simulink model "bluetooth"  (R2020a)
settings: Solver=FixedStepAuto  StartTime=0.0  StopTime=10.0  RelTol=1e-3
undefined symbols (not defined in the file): BC, Ci, Ri, tau1
libraries: androiduilib x12, simulink x5, androidcommunicationlib x2, dspswit3 x2
settings Model: Creator=luisi  LastModifiedBy=luisi
settings OptimizationCC: EnhancedBackFolding=on  PassReuseOutputArgsAs=Individual arguments  ZeroExternalMemoryAtStartup=off  ZeroInternalMemoryAtStartup=off  MaxStackSize=64  OptimizeBlockOrder=speed  DifferentSizesBufferReuse=on  OptimizationCustomize=off  EfficientTunableParamExpr=on
settings DebuggingCC: ParameterTunabilityLossMsg=error
settings HardwareCC: ProdBitPerPointer=32  ProdBitPerSizeT=32  ProdBitPerPtrDiffT=32  ProdLargestAtomicInteger=Long  ProdLargestAtomicFloat=Double  ProdWordSize=32  ProdHWDeviceType=ARM Compatible->ARM Cortex
settings SFSimCC: MATLABDynamicMemAlloc=off
settings RTWCC: SystemTargetFile=ert.tlc  HardwareBoard=Android Device  TemplateMakefile=ert_default_tmf  RTWVerbose=off  Toolchain=Android SDK/NDK Tools
settings CodeAppCC: ForceParamTrailComments=on  IgnoreCustomStorageClasses=off  OperatorAnnotations=on  SimulinkDataObjDesc=on  SFDataObjDesc=on  InsertBlockDesc=on
settings ERTTargetCC: SupportContinuousTime=on  SupportVariableSizeSignals=on  ExtModeMexArgs='192.168.0.149'

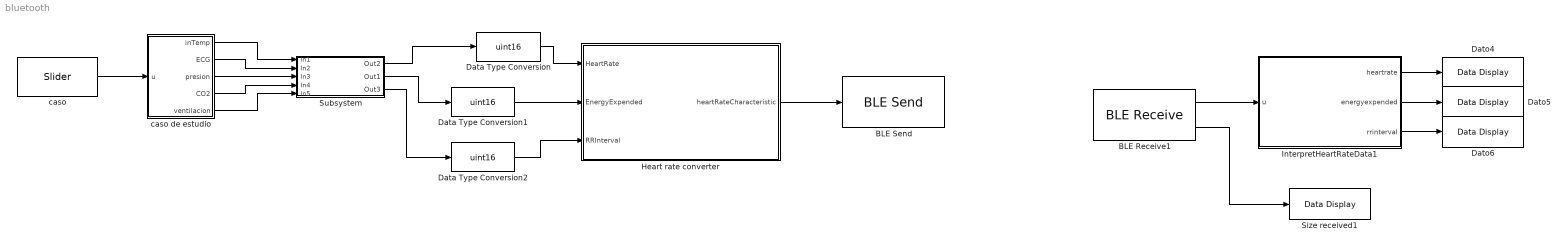
== system bluetooth ==
  BLE Receive1 : androidcommunicationlib/BLE Receive  DeviceMode=Central (Client)  BluetoothAddress=75:BC:6F:E0:E0:E0  CharUUID=00002a37-0000-1000-8000-00805f9b34fb  ServiceUUID=0000180d-0000-1000-8000-00805f9b34fb  device=RedmiMama  character="Heart Rate\\Heart Rate  Measurement"  CustomService=off  ServiceName=Heart Rate  CharacteristicName="Heart Rate  Measurement"  CustomServiceUUID=<Enter Service UUID>  CustomCharUUID=<Enter Characteristic UUID>  DataSize=7  SampleTime=0.1  charseruuid=00001801-0000-1000-8000-00805f9b34fb\00002a05-0000-1000-8000-00805f9b34fb  seruuid=00001810-0000-1000-8000-00805f9b34fb  PeripheralService=0000180d-0000-1000-8000-00805f9b34fb  PeripheralCharacteristic=00002a37-0000-1000-8000-00805f9b34fb  chruuid=00002a37-0000-1000-8000-00805f9b34fb  BLEId=bluetooth/BLE_Receive1  Devicename=RedmiMama  IsCustomService=0
      settings: SourceProductBaseCode=ANDROID
  BLE Send : androidcommunicationlib/BLE Send  DeviceMode=Peripheral (Server)  BluetoothAddress=75:BC:6F:E0:E0:E0  CharUUID=00002a05-0000-1000-8000-00805f9b34fb  ServiceUUID=00001801-0000-1000-8000-00805f9b34fb  device=RedmiMama  character=Generic Attribute\Service Changed  CustomService=off  ServiceName=Heart Rate  CharacteristicName="Heart Rate  Measurement"  CustomServiceUUID=<Enter Service UUID>  CustomCharUUID=<Enter Characteristic UUID>  charseruuid=00001801-0000-1000-8000-00805f9b34fb\00002a05-0000-1000-8000-00805f9b34fb  seruuid=00001810-0000-1000-8000-00805f9b34fb  chruuid=00002a37-0000-1000-8000-00805f9b34fb  PeripheralService=0000180d-0000-1000-8000-00805f9b34fb  PeripheralCharacteristic=00002a37-0000-1000-8000-00805f9b34fb  BLEId=bluetooth/BLE_Send  Devicename=RedmiMama  IsCustomService=0  Size=-1
      settings: SourceProductBaseCode=ANDROID
  Data Type Conversion : DataTypeConversion  OutDataTypeStr=uint16
  Data Type Conversion1 : DataTypeConversion  OutDataTypeStr=uint16
  Data Type Conversion2 : DataTypeConversion  OutDataTypeStr=uint16
  Dato4 : androiduilib/Data Display  DataDisplayId=bluetooth/Dato4  Format=Float  Precision=6  SimulateUsing=Code generation  blockPlatform=Android
      settings: SourceProductBaseCode=ANDROID
  Dato5 : androiduilib/Data Display  DataDisplayId=bluetooth/Dato5  Format=Float  Precision=6  SimulateUsing=Code generation  blockPlatform=Android
      settings: SourceProductBaseCode=ANDROID
  Dato6 : androiduilib/Data Display  DataDisplayId=bluetooth/Dato6  Format=Float  Precision=6  SimulateUsing=Code generation  blockPlatform=Android
      settings: SourceProductBaseCode=ANDROID
  Heart rate converter : MATLAB Function  TreatAsAtomicUnit=on
  InterpretHeartRateData1 : MATLAB Function  TreatAsAtomicUnit=on
  Size received1 : androiduilib/Data Display  DataDisplayId=bluetooth/Size_received1  Format=Float  Precision=6  SimulateUsing=Code generation  blockPlatform=Android
      settings: SourceProductBaseCode=ANDROID
  Subsystem : Subsystem
  caso : androiduilib/Slider  Min=0  Value=0  Max=2  Resolution=1  SliderId=bluetooth/caso  SampleTime=0.01  BlockPlatform=Android
      settings: SourceProductBaseCode=ANDROID
  caso de estudio : MATLAB Function  TreatAsAtomicUnit=on
  wires:
  Data Type Conversion2/1 -> Heart rate converter/3(RRInterval)
  Heart rate converter/1(heartRateCharacteristic) -> BLE Send/1
  Data Type Conversion/1 -> Heart rate converter/1(HeartRate)
  Data Type Conversion1/1 -> Heart rate converter/2(EnergyExpended)
  Subsystem/1(Out2) -> Data Type Conversion/1
  Subsystem/2(Out1) -> Data Type Conversion1/1
  Subsystem/3(Out3) -> Data Type Conversion2/1
  InterpretHeartRateData1/1(heartrate) -> Dato4/1
  BLE Receive1/2 -> Size received1/1
  InterpretHeartRateData1/2(energyexpended) -> Dato5/1
  InterpretHeartRateData1/3(rrinterval) -> Dato6/1
  BLE Receive1/1 -> InterpretHeartRateData1/1(u)
  caso de estudio/3(presion) -> Subsystem/3(In3)
  caso/1 -> caso de estudio/1(u)
  caso de estudio/4(CO2) -> Subsystem/4(In4)
  caso de estudio/2(ECG) -> Subsystem/2(In2)
  caso de estudio/5(ventilacion) -> Subsystem/5(In5)
  caso de estudio/1(inTemp) -> Subsystem/1(In1)

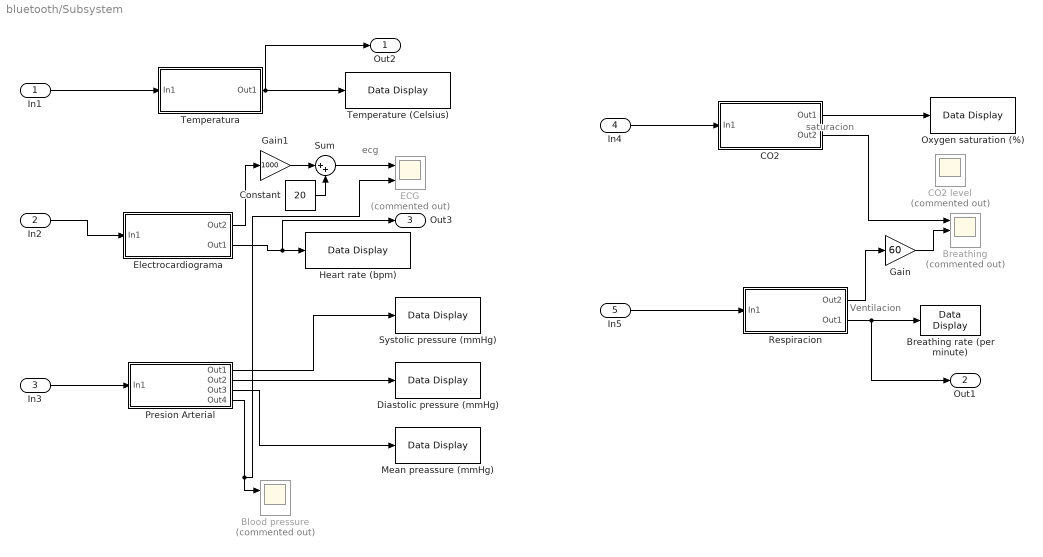
== system bluetooth/Subsystem ==
  note: ecg
  note: saturacion
  note: Ventilacion
  In1 : Inport
  In2 : Inport  Port=2
  In3 : Inport  Port=3
  In4 : Inport  Port=4
  In5 : Inport  Port=5
  Blood pressure : Scope  Commented=on  NumInputPorts=2
  Breathing : Scope  Commented=on  NumInputPorts=3
  Breathing rate (per minute) : androiduilib/Data Display  DataDisplayId=bluetooth/Subsystem/Breathing_rate_(per_minute)  Format=Integer  Precision=6  SimulateUsing=Code generation  blockPlatform=Android
      settings: SourceProductBaseCode=ANDROID
  CO2 : Subsystem
  "CO2 level " : Scope  Commented=on
  Constant : Constant  Value=20
  Diastolic pressure (mmHg) : androiduilib/Data Display  DataDisplayId=bluetooth/Subsystem/Diastolic_pressure_(mmHg)  Format=Integer  Precision=6  SimulateUsing=Code generation  blockPlatform=Android
      settings: SourceProductBaseCode=ANDROID
  ECG : Scope  Commented=on  NumInputPorts=2
      settings: AttributesFormatString=%<AxesScaling>
  Electrocardiograma : Subsystem
  Gain : Gain  Gain=60
  Gain1 : Gain  Gain=1000
  Heart rate (bpm) : androiduilib/Data Display  DataDisplayId=bluetooth/Subsystem/Heart_rate_(bpm)  Format=Float  Precision=6  SimulateUsing=Code generation  blockPlatform=Android
      settings: SourceProductBaseCode=ANDROID
  Mean preassure (mmHg) : androiduilib/Data Display  DataDisplayId=bluetooth/Subsystem/Mean_preassure_(mmHg)  Format=Integer  Precision=6  SimulateUsing=Code generation  blockPlatform=Android
      settings: SourceProductBaseCode=ANDROID
  Oxygen saturation (%) : androiduilib/Data Display  DataDisplayId=bluetooth/Subsystem/Oxygen_saturation_(%)  Format=Integer  Precision=6  SimulateUsing=Code generation  blockPlatform=Android
      settings: SourceProductBaseCode=ANDROID
  Presion Arterial : Subsystem
  Respiracion : Subsystem
  Sum : Sum  Inputs=|++
  Systolic pressure (mmHg) : androiduilib/Data Display  DataDisplayId=bluetooth/Subsystem/Systolic_pressure_(mmHg)  Format=Integer  Precision=6  SimulateUsing=Code generation  blockPlatform=Android
      settings: SourceProductBaseCode=ANDROID
  Temperatura : Subsystem
  Temperature (Celsius) : androiduilib/Data Display  DataDisplayId=bluetooth/Subsystem/Temperature_(Celsius)  Format=Float  Precision=1  SimulateUsing=Code generation  blockPlatform=Android
      settings: SourceProductBaseCode=ANDROID
  Out2 : Outport
  Out1 : Outport  Port=2
  Out3 : Outport  Port=3
  wires:
  In1/1 -> Temperatura/1(In1)
  In2/1 -> Electrocardiograma/1(In1)
  Temperatura/1(Out1) -> Out2/1, Temperature (Celsius)/1
  Presion Arterial/2(Out2) -> Diastolic pressure (mmHg)/1
  Presion Arterial/3(Out3) -> Mean preassure (mmHg)/1
  Presion Arterial/1(Out1) -> Systolic pressure (mmHg)/1
  In5/1 -> Respiracion/1(In1)
  In3/1 -> Presion Arterial/1(In1)
  In4/1 -> CO2/1(In1)
  CO2/1(Out1) -> Oxygen saturation (%)/1
  Respiracion/2(Out1) -> Out1/1, Breathing rate (per minute)/1
  Electrocardiograma/2(Out1) -> Out3/1, Heart rate (bpm)/1
  CO2/2(Out2) -> Breathing/1
  Respiracion/1(Out2) -> Gain/1
  Gain/1 -> Breathing/2
  Presion Arterial/4(Out4) -> ECG/2, Blood pressure/1
  Electrocardiograma/1(Out2) -> Gain1/1
  Gain1/1 -> Sum/1
  Constant/1 -> Sum/2
  Sum/1 -> ECG/1

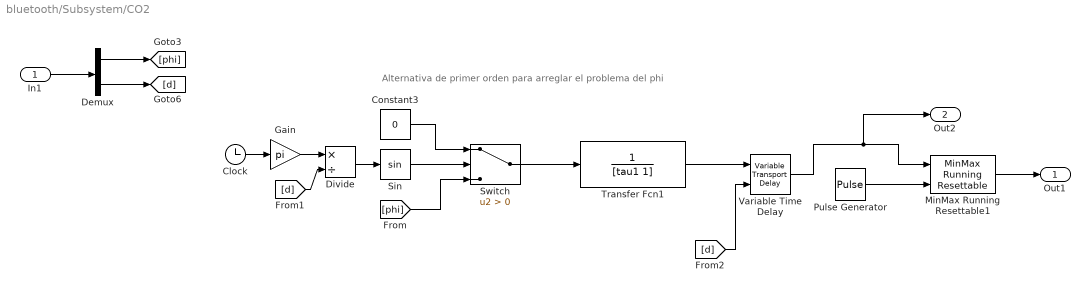
== system bluetooth/Subsystem/CO2 ==
  note: Alternativa de primer orden para arreglar el problema del phi
  In1 : Inport
  Clock : Clock
  Constant3 : Constant  Value=0
  Demux : Demux  Outputs=2
  Divide : Product  Inputs=*/
  Gain : Gain  Gain=pi
  MinMax Running Resettable1 : simulink/Math Operations/MinMax Running Resettable  Function=max  vinit=0
  Pulse Generator : DiscretePulseGenerator  PulseType=Time based  Period=4  PulseWidth=5  PhaseDelay=0.01
  Sin : Trigonometry
  Switch : Switch  Criteria=u2 > Threshold
  Transfer Fcn1 : TransferFcn  Denominator=[tau1 1]
  Variable Time Delay : VariableTransportDelay  MaximumDelay=10
  Out1 : Outport
  Out2 : Outport  Port=2
  wires:
  In1/1 -> Demux/1
  Demux/1 -> [phi]
  Switch/1 -> Transfer Fcn1/1
  Sin/1 -> Switch/2
  [phi] -> Switch/3
  Constant3/1 -> Switch/1
  Demux/2 -> [d]
  Clock/1 -> Gain/1
  Gain/1 -> Divide/1
  Divide/1 -> Sin/1
  [d] -> Divide/2
  MinMax Running Resettable1/1 -> Out1/1
  Pulse Generator/1 -> MinMax Running Resettable1/2
  Transfer Fcn1/1 -> Variable Time Delay/1
  Variable Time Delay/1 -> Out2/1, MinMax Running Resettable1/1
  [d] -> Variable Time Delay/2

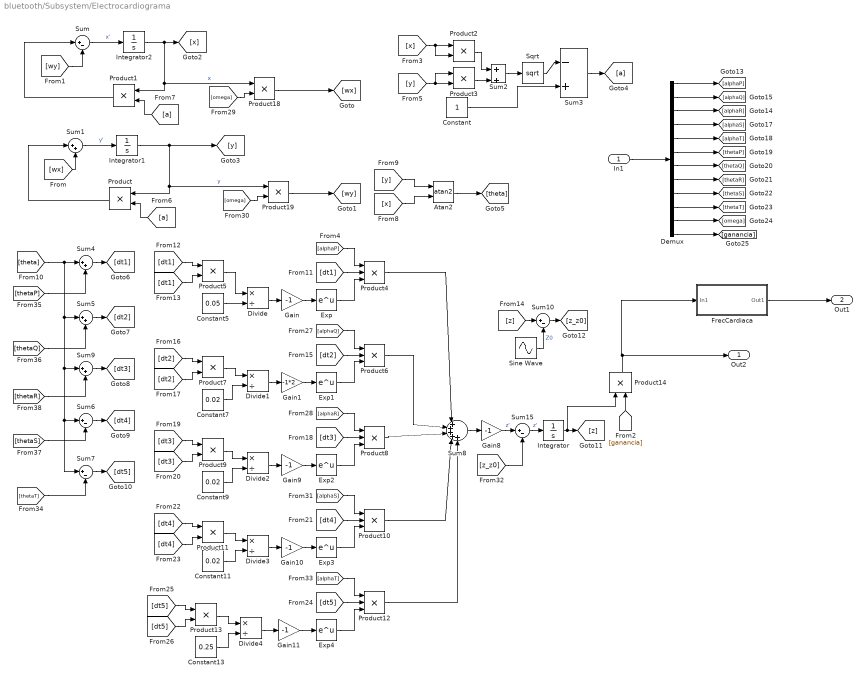
== system bluetooth/Subsystem/Electrocardiograma ==
  In1 : Inport
  Atan2 : Trigonometry  Operator=atan2
  Constant : Constant
  Constant11 : Constant  Value=0.02
  Constant13 : Constant  Value=0.25
  Constant5 : Constant  Value=0.05
  Constant7 : Constant  Value=0.02
  Constant9 : Constant  Value=0.02
  Demux : Demux  Outputs=12
  Divide{,1..4} (5 alike) : Product  Inputs=*/
  Exp{,1..4} (5 alike) : Math  SaturateOnIntegerOverflow=on
  FrecCardiaca : Subsystem
  Gain{,8..11} (5 alike) : Gain  Gain=-1
  Gain1 : Gain  Gain=-1*2
  Integrator : Integrator  InitialCondition=1000
  Integrator1 : Integrator
  Integrator2 : Integrator  InitialCondition=2
  Product{,1..3,5,7,9,11,13..14,18..19} (12 alike) : Product
  Product{4,6,8,10,12} (5 alike) : Product  Inputs=3
  Sine Wave : Sin  Amplitude=0.15e-3  Frequency=0.25  SampleTime=0
  Sqrt : Sqrt  SaturateOnIntegerOverflow=on
  Sum{,6..7,10,15} (5 alike) : Sum  Inputs=|+-
  Sum{1..2,4..5,9} (5 alike) : Sum  Inputs=|++
  Sum3 : Sum  Inputs=|-+
  Sum8 : Sum  Inputs=|+++++
  Out2 : Outport
  Out1 : Outport  Port=2
  wires:
  [dt2] -> Product6/2
  Product4/1 -> Sum8/1
  [x] -> Atan2/2
  Product3/1 -> Sum2/2
  [y] -> Atan2/1
  FrecCardiaca/1(Out1) -> Out1/1
  Product/1 -> Sum1/1
  Product5/1 -> Divide/1
  [dt2] -> Product7/2
  Gain/1 -> Exp/1
  Product1/1 -> Sum/1
  Constant/1 -> Sum3/2
  Divide1/1 -> Gain1/1
  Exp4/1 -> Product12/3
  Exp3/1 -> Product10/3
  Gain11/1 -> Exp4/1
  Exp/1 -> Product4/3
  [alphaT] -> Product12/1
  Constant11/1 -> Divide3/2
  Divide2/1 -> Gain9/1
  [dt1] -> Product4/2
  Product18/1 -> [wx]
  Sum2/1 -> Sqrt/1
  [a] -> Product1/2
  [thetaP] -> Sum4/2
  Product8/1 -> Sum8/3
  Exp2/1 -> Product8/3
  Product11/1 -> Divide3/1
  [dt3] -> Product9/2
  Integrator1/1 -> [y], Product19/1, Product/1  "y"
  Constant5/1 -> Divide/2
  Product7/1 -> Divide1/1
  [dt4] -> Product11/1
  Sqrt/1 -> Sum3/1
  Product13/1 -> Divide4/1
  Gain10/1 -> Exp3/1
  [dt1] -> Product5/1
  Gain1/1 -> Exp1/1
  [dt5] -> Product13/2
  [dt4] -> Product11/2
  [dt1] -> Product5/2
  Constant9/1 -> Divide2/2
  [dt5] -> Product12/2
  Divide/1 -> Gain/1
  Divide4/1 -> Gain11/1
  [dt5] -> Product13/1
  Product12/1 -> Sum8/5
  Product6/1 -> Sum8/2
  Constant13/1 -> Divide4/2
  Product10/1 -> Sum8/4
  Sum5/1 -> [dt2]
  [dt4] -> Product10/2
  Sine Wave/1 -> Sum10/2  "Z0"
  Sum6/1 -> [dt4]
  Sum1/1 -> Integrator1/1  "y'"
  [dt3] -> Product9/1
  Atan2/1 -> [theta]
  [omega] -> Product19/2
  Sum7/1 -> [dt5]
  Sum10/1 -> [z_z0]
  Gain8/1 -> Sum15/1  "z'"
  Integrator/1 -> Product14/1, [z]
  [dt3] -> Product8/2
  [theta] -> Sum7/1, Sum6/1, Sum9/1, Sum5/1, Sum4/1
  [z_z0] -> Sum15/2
  [a] -> Product/2
  Integrator2/1 -> [x], Product1/1, Product18/1  "x"
  Exp1/1 -> Product6/3
  [thetaS] -> Sum6/2
  Sum4/1 -> [dt1]
  [alphaP] -> Product4/1
  Sum15/1 -> Integrator/1  "z'"
  Product19/1 -> [wy]
  Sum/1 -> Integrator2/1  "x'"
  [wx] -> Sum1/2
  [thetaT] -> Sum7/2
  [y] -> Product3/1, Product3/2
  [wy] -> Sum/2
  [thetaQ] -> Sum5/2
  Product9/1 -> Divide2/1
  Constant7/1 -> Divide1/2
  Sum3/1 -> [a]
  [x] -> Product2/2, Product2/1
  [dt2] -> Product7/1
  [z] -> Sum10/1
  Gain9/1 -> Exp2/1
  [omega] -> Product18/2
  Product2/1 -> Sum2/1
  Product14/1 -> FrecCardiaca/1(In1), Out2/1
  Divide3/1 -> Gain10/1
  Sum8/1 -> Gain8/1
  In1/1 -> Demux/1
  Demux/1 -> [alphaP]
  Demux/2 -> [alphaQ]
  Demux/3 -> [alphaR]
  Demux/4 -> [alphaS]
  Demux/5 -> [alphaT]
  Demux/6 -> [thetaP]
  Demux/7 -> [thetaQ]
  Demux/8 -> [thetaR]
  Demux/9 -> [thetaS]
  Demux/10 -> [thetaT]
  Demux/11 -> [omega]
  Demux/12 -> [ganancia]
  [ganancia] -> Product14/2
  [alphaS] -> Product10/1
  [alphaR] -> Product8/1
  [alphaQ] -> Product6/1
  Sum9/1 -> [dt3]
  [thetaR] -> Sum9/2

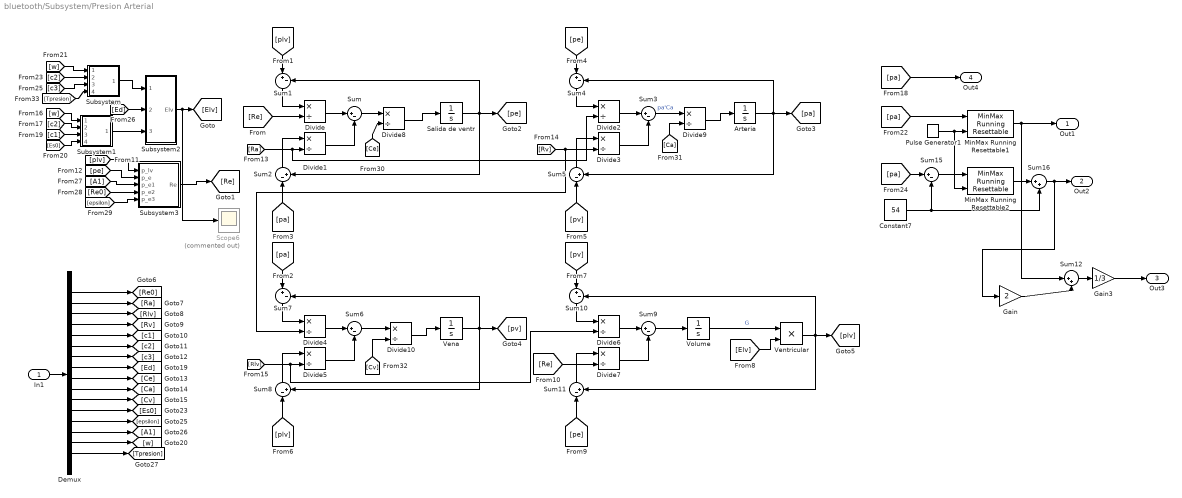
== system bluetooth/Subsystem/Presion Arterial ==
  In1 : Inport
  Arteria : Integrator  InitialCondition=70
  Constant7 : Constant  Value=54
  Demux : Demux  Outputs=16
  Divide{,1..10} (11 alike) : Product  Inputs=*/
  Gain : Gain  Gain=2
  Gain3 : Gain  Gain=1/3
  MinMax Running Resettable1 : simulink/Math Operations/MinMax Running Resettable  Function=max  vinit=40
  MinMax Running Resettable2 : simulink/Math Operations/MinMax Running Resettable  Function=min  vinit=0.0
  Pulse Generator1 : DiscretePulseGenerator  PulseType=Time based  Period=8  PulseWidth=5
  Salida de ventr : Integrator  InitialCondition=49.896
  Scope6 : Scope  Commented=on
  Subsystem : Subsystem
  Subsystem1 : Subsystem
  Subsystem2 : Subsystem
  Subsystem3 : Subsystem
  Sum{,1,3..4,6..7,9..10,15} (9 alike) : Sum  Inputs=|+-
  Sum{2,5,8,11} (4 alike) : Sum  Inputs=|-+
  Sum12 : Sum  Inputs=|++
  Sum16 : Sum  Inputs=|++
  Vena : Integrator  InitialCondition=16.628
  Ventricular : Product
  Volume : Integrator  InitialCondition=49.714/0.0655
  Out1 : Outport
  Out2 : Outport  Port=2
  Out3 : Outport  Port=3
  Out4 : Outport  Port=4
  wires:
  Gain3/1 -> Out3/1
  Sum16/1 -> Gain/1, Out2/1
  MinMax Running Resettable2/1 -> Sum16/1
  Sum3/1 -> Divide9/1  "pa'Ca"
  [pa] -> MinMax Running Resettable1/1
  Sum10/1 -> Divide6/1
  MinMax Running Resettable1/1 -> Sum12/1, Out1/1
  Subsystem2/1(Elv) -> Scope6/1, [Elv]
  Constant7/1 -> Sum16/2, Sum15/2
  Salida de ventr/1 -> [pe], Sum2/2, Sum1/2
  [pa] -> Sum15/1
  Divide6/1 -> Sum9/1
  Pulse Generator1/1 -> MinMax Running Resettable2/2, MinMax Running Resettable1/2
  [Elv] -> Ventricular/2
  [pa] -> Out4/1
  Divide8/1 -> Salida de ventr/1
  [Re] -> Divide/2
  [Rv] -> Divide4/2, Divide3/2
  Sum5/1 -> Divide3/1
  [plv] -> Subsystem3/1(p_lv)
  Divide/1 -> Sum/1
  [plv] -> Sum1/1
  [pv] -> Sum10/1
  Ventricular/1 -> Sum10/2, [plv], Sum11/2
  Sum15/1 -> MinMax Running Resettable2/1
  [pe] -> Sum4/1
  [pe] -> Subsystem3/2(p_e)
  Sum9/1 -> Volume/1
  [plv] -> Sum8/1
  Divide10/1 -> Vena/1
  [pv] -> Sum5/1
  Divide7/1 -> Sum9/2
  [Rlv] -> Divide6/2, Divide5/2
  Divide9/1 -> Arteria/1
  Sum8/1 -> Divide5/1
  Sum11/1 -> Divide7/1
  Divide2/1 -> Sum3/1
  [pe] -> Sum11/1
  [pa] -> Sum7/1
  Sum7/1 -> Divide4/1
  Vena/1 -> [pv], Sum8/2, Sum7/2
  Divide3/1 -> Sum3/2
  Sum6/1 -> Divide10/1
  Volume/1 -> Ventricular/1  "G"
  Divide5/1 -> Sum6/2
  Divide4/1 -> Sum6/1
  Arteria/1 -> Sum5/2, Sum4/2, [pa]
  [pa] -> Sum2/1
  [Re] -> Divide7/2
  Sum2/1 -> Divide1/1
  Sum1/1 -> Divide/1
  Sum/1 -> Divide8/1
  Sum4/1 -> Divide2/1
  Subsystem3/1(Re) -> [Re]
  Subsystem/1(alpha_t) -> Subsystem2/1(alpha)
  Subsystem1/1(E_s) -> Subsystem2/3(E_s)
  Divide1/1 -> Sum/2
  [Ra] -> Divide2/2, Divide1/2
  In1/1 -> Demux/1
  [w] -> Subsystem1/1(In1)
  [c2] -> Subsystem1/2(In2)
  [c1] -> Subsystem1/3(In3)
  [Es0] -> Subsystem1/4(In4)
  [w] -> Subsystem/1(In1)
  [c2] -> Subsystem/2(In2)
  [c3] -> Subsystem/3(In3)
  [Ed] -> Subsystem2/2(In2)
  [A1] -> Subsystem3/3(p_e1)
  [Re0] -> Subsystem3/4(p_e2)
  [epsilon] -> Subsystem3/5(p_e3)
  [Ce] -> Divide8/2
  [Ca] -> Divide9/2
  [Cv] -> Divide10/2
  Demux/1 -> [Re0]
  Demux/2 -> [Ra]
  Demux/3 -> [Rlv]
  Demux/4 -> [Rv]
  Demux/5 -> [c1]
  Demux/6 -> [c2]
  Demux/7 -> [c3]
  Demux/8 -> [Ed]
  Demux/9 -> [Ce]
  Demux/10 -> [Ca]
  Demux/11 -> [Cv]
  Demux/12 -> [Es0]
  Demux/13 -> [epsilon]
  Demux/14 -> [A1]
  Demux/15 -> [w]
  [Tpresion] -> Subsystem/4(In4)
  Demux/16 -> [Tpresion]
  Sum12/1 -> Gain3/1
  Gain/1 -> Sum12/2

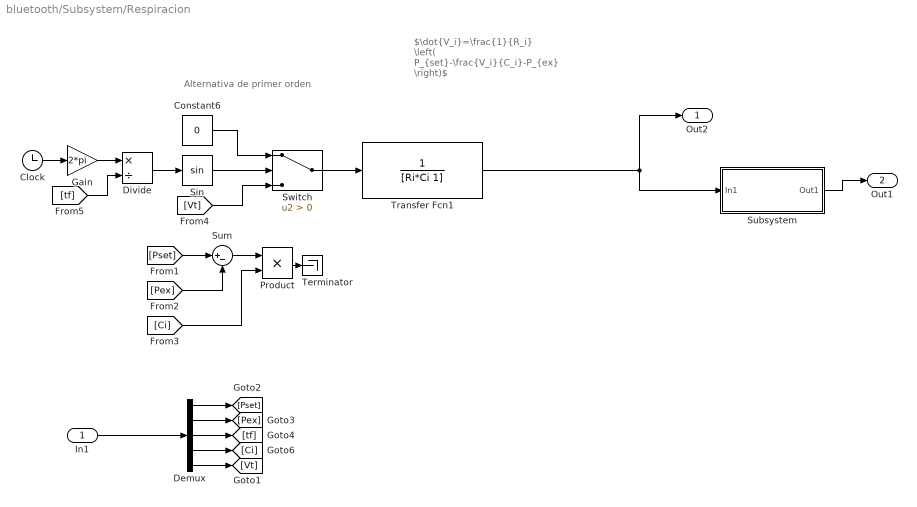
== system bluetooth/Subsystem/Respiracion ==
  note: $\dot{V_i}=\frac{1}{R_i} \left( P_{set}-\frac{V_i}{C_i}-P_{ex} \right)$
  note: Alternativa de primer orden
  In1 : Inport
  Clock : Clock
  Constant6 : Constant  Value=0
  Demux : Demux  Outputs=5
  Divide : Product  Inputs=*/
  Gain : Gain  Gain=2*pi
  Product : Product
  Sin : Trigonometry
  Subsystem : Subsystem
  Sum : Sum  Inputs=|+-
  Switch : Switch  Criteria=u2 > Threshold
  Terminator : Terminator
  Transfer Fcn1 : TransferFcn  Denominator=[Ri*Ci 1]
  Out2 : Outport
  Out1 : Outport  Port=2
  wires:
  Subsystem/1(Out1) -> Out1/1
  Demux/1 -> [Pset]
  Demux/2 -> [Pex]
  Demux/3 -> [tf]
  In1/1 -> Demux/1
  Transfer Fcn1/1 -> Out2/1, Subsystem/1(In1)
  [Ci] -> Product/2
  Switch/1 -> Transfer Fcn1/1
  Sum/1 -> Product/1
  Product/1 -> Terminator/1
  [Vt] -> Switch/3
  Sin/1 -> Switch/2
  [Pex] -> Sum/2
  Constant6/1 -> Switch/1
  [Pset] -> Sum/1
  Clock/1 -> Gain/1
  Gain/1 -> Divide/1
  [tf] -> Divide/2
  Divide/1 -> Sin/1
  Demux/4 -> [Ci]
  Demux/5 -> [Vt]

== system bluetooth/Subsystem/Temperatura ==
  In1 : Inport
  Data Type Conversion : DataTypeConversion
  Sine Wave : Sin  Amplitude=0.005  Frequency=20  SampleTime=0
  Sum : Sum  Inputs=|++
  Transfer Fcn : TransferFcn  Numerator=36.8  Denominator=[0.4 1]
  Out1 : Outport
  wires:
  Data Type Conversion/1 -> Transfer Fcn/1
  Transfer Fcn/1 -> Out1/1
  In1/1 -> Sum/1
  Sine Wave/1 -> Sum/2
  Sum/1 -> Data Type Conversion/1

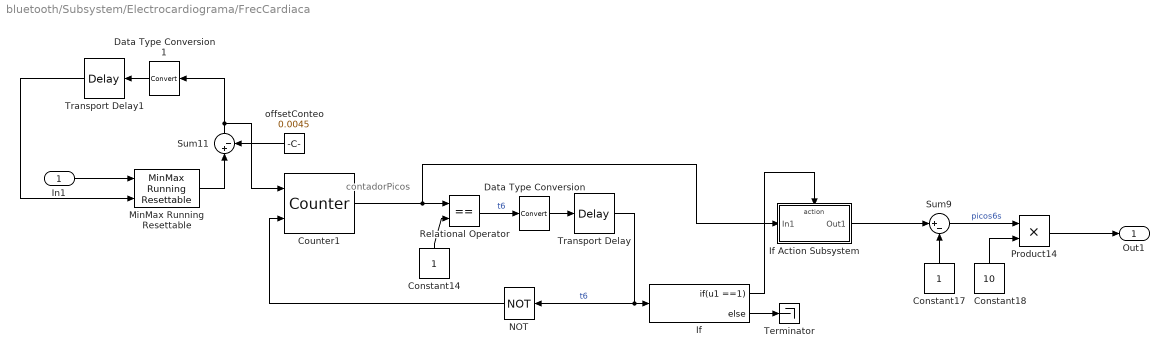
== system bluetooth/Subsystem/Electrocardiograma/FrecCardiaca ==
  note: contadorPicos
  In1 : Inport
  Constant14 : Constant
  Constant17 : Constant
  Constant18 : Constant  Value=10
  Counter1 : dspswit3/Counter  Direction=Up  CountEvent=Rising edge  CounterSize=User defined  MaxCount=100  InitialCount=0  Output=Count  HitValue=32  ResetInput=on  SamplesPerFrame=1  Ts=1  CntDtype=double  HitDtype=Logical
  Data Type Conversion : DataTypeConversion
  Data Type Conversion1 : DataTypeConversion
  If : If  IfExpression=u1 ==1
  If Action Subsystem : Subsystem  TreatAsAtomicUnit=on
  MinMax Running Resettable : simulink/Math Operations/MinMax Running Resettable  Function=max  vinit=0.0045
  NOT : Logic  Operator=NOT  IconShape=distinctive  AllPortsSameDT=off  OutDataTypeStr=boolean
  Product14 : Product
  Relational Operator : RelationalOperator  Operator===  OutDataTypeStr=boolean  RndMeth=Simplest
  Sum11 : Sum  Inputs=|+-
  Sum9 : Sum  Inputs=|+-
  Terminator : Terminator
  Transport Delay : TransportDelay  DelayTime=6
  Transport Delay1 : TransportDelay  DelayTime=0.16
  offsetConteo : Constant  Value=0.0045
  Out1 : Outport
  wires:
  NOT/1 -> Counter1/2
  Sum9/1 -> Product14/1  "picos6s"
  If/2 -> Terminator/1
  Product14/1 -> Out1/1
  If Action Subsystem/1(Out1) -> Sum9/1
  If/1 -> If Action Subsystem/Action
  Transport Delay/1 -> NOT/1, If/1  "t6"
  Constant17/1 -> Sum9/2
  Constant14/1 -> Relational Operator/2
  In1/1 -> MinMax Running Resettable/1
  Counter1/1 -> If Action Subsystem/1(In1), Relational Operator/1
  MinMax Running Resettable/1 -> Sum11/1
  offsetConteo/1 -> Sum11/2
  Constant18/1 -> Product14/2
  Transport Delay1/1 -> MinMax Running Resettable/2
  Sum11/1 -> Data Type Conversion1/1, Counter1/1
  Relational Operator/1 -> Data Type Conversion/1  "t6"
  Data Type Conversion/1 -> Transport Delay/1
  Data Type Conversion1/1 -> Transport Delay1/1

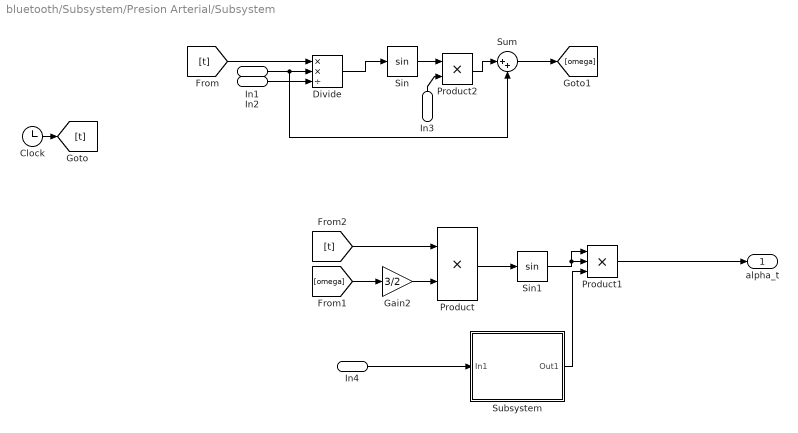
== system bluetooth/Subsystem/Presion Arterial/Subsystem ==
  In1 : Inport
  In2 : Inport  Port=2
  In3 : Inport  Port=3
  In4 : Inport  Port=4
  Clock : Clock
  Divide : Product  Inputs=**/
  Gain2 : Gain  Gain=3/2
  Product : Product
  Product1 : Product  Inputs=3
  Product2 : Product
  Sin : Trigonometry
  Sin1 : Trigonometry
  Subsystem : Subsystem
  Sum : Sum  Inputs=|++
  alpha_t : Outport
  wires:
  Clock/1 -> [t]
  [t] -> Divide/1
  Divide/1 -> Sin/1
  Sin/1 -> Product2/1
  Product2/1 -> Sum/1
  In1/1 -> Sum/2, Divide/2
  Sum/1 -> [omega]
  [t] -> Product/1
  [omega] -> Gain2/1
  Product/1 -> Sin1/1
  Sin1/1 -> Product1/1, Product1/2
  Product1/1 -> alpha_t/1
  Gain2/1 -> Product/2
  Subsystem/1(Out1) -> Product1/3
  In2/1 -> Divide/3
  In3/1 -> Product2/2
  In4/1 -> Subsystem/1(In1)

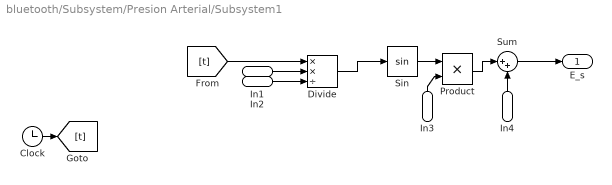
== system bluetooth/Subsystem/Presion Arterial/Subsystem1 ==
  In1 : Inport
  In2 : Inport  Port=2
  In3 : Inport  Port=3
  In4 : Inport  Port=4
  Clock : Clock
  Divide : Product  Inputs=**/
  Product : Product
  Sin : Trigonometry
  Sum : Sum  Inputs=|++
  E_s : Outport
  wires:
  Sum/1 -> E_s/1
  In4/1 -> Sum/2
  Product/1 -> Sum/1
  Sin/1 -> Product/1
  Divide/1 -> Sin/1
  [t] -> Divide/1
  Clock/1 -> [t]
  In2/1 -> Divide/3
  In1/1 -> Divide/2
  In3/1 -> Product/2

== system bluetooth/Subsystem/Presion Arterial/Subsystem2 ==
  alpha : Inport
  In2 : Inport  Port=2
  E_s : Inport  Port=3
  Product : Product
  Sum : Sum
  Sum1 : Sum  Inputs=-+
  Elv : Outport
  wires:
  In2/1 -> Sum1/1, Sum/1
  E_s/1 -> Sum1/2
  alpha/1 -> Product/2
  Sum1/1 -> Product/1
  Product/1 -> Sum/2
  Sum/1 -> Elv/1

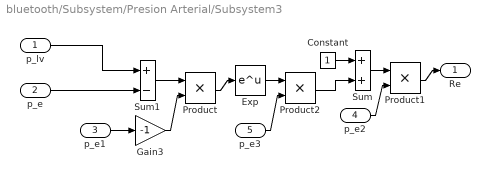
== system bluetooth/Subsystem/Presion Arterial/Subsystem3 ==
  p_lv : Inport
  p_e : Inport  Port=2
  p_e1 : Inport  Port=3
  p_e2 : Inport  Port=4
  p_e3 : Inport  Port=5
  Constant : Constant
  Exp : Math  SaturateOnIntegerOverflow=on
  Gain3 : Gain  Gain=-1
  Product : Product
  Product1 : Product
  Product2 : Product
  Sum : Sum
  Sum1 : Sum  Inputs=+-
  Re : Outport
  wires:
  Sum/1 -> Product1/1
  Product1/1 -> Re/1
  Constant/1 -> Sum/1
  Product2/1 -> Sum/2
  Exp/1 -> Product2/1
  p_lv/1 -> Sum1/1
  p_e/1 -> Sum1/2
  Product/1 -> Exp/1
  Sum1/1 -> Product/1
  p_e1/1 -> Gain3/1
  Gain3/1 -> Product/2
  p_e2/1 -> Product1/2
  p_e3/1 -> Product2/2

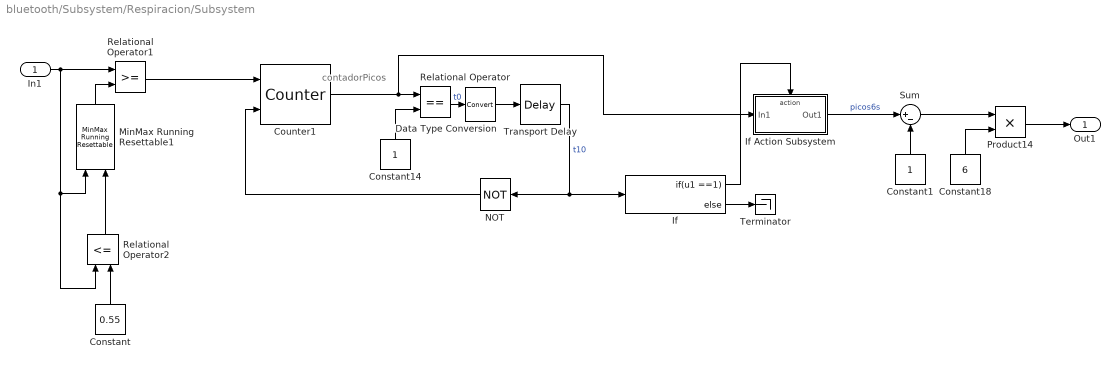
== system bluetooth/Subsystem/Respiracion/Subsystem ==
  note: contadorPicos
  In1 : Inport
  Constant : Constant  Value=0.55
  Constant1 : Constant
  Constant14 : Constant
  Constant18 : Constant  Value=6
  Counter1 : dspswit3/Counter  Direction=Up  CountEvent=Rising edge  CounterSize=User defined  MaxCount=100  InitialCount=0  Output=Count  HitValue=32  ResetInput=on  SamplesPerFrame=1  Ts=1  CntDtype=double  HitDtype=Logical
  Data Type Conversion : DataTypeConversion
  If : If  IfExpression=u1 ==1
  If Action Subsystem : Subsystem  TreatAsAtomicUnit=on
  MinMax Running Resettable1 : simulink/Math Operations/MinMax Running Resettable  Function=max  vinit=0.55
  NOT : Logic  Operator=NOT  IconShape=distinctive  AllPortsSameDT=off  OutDataTypeStr=boolean
  Product14 : Product
  Relational Operator : RelationalOperator  Operator===  OutDataTypeStr=boolean  RndMeth=Simplest
  Relational Operator1 : RelationalOperator  OutDataTypeStr=boolean  RndMeth=Simplest
  Relational Operator2 : RelationalOperator  Operator=<=  OutDataTypeStr=boolean  RndMeth=Simplest
  Sum : Sum  Inputs=|+-
  Terminator : Terminator
  Transport Delay : TransportDelay  DelayTime=10
  Out1 : Outport
  wires:
  Relational Operator1/1 -> Counter1/1
  Product14/1 -> Out1/1
  If/2 -> Terminator/1
  Constant18/1 -> Product14/2
  Transport Delay/1 -> NOT/1, If/1  "t10"
  NOT/1 -> Counter1/2
  Counter1/1 -> If Action Subsystem/1(In1), Relational Operator/1
  If/1 -> If Action Subsystem/Action
  Constant14/1 -> Relational Operator/2
  MinMax Running Resettable1/1 -> Relational Operator1/2
  Relational Operator/1 -> Data Type Conversion/1  "t0"
  Data Type Conversion/1 -> Transport Delay/1
  In1/1 -> Relational Operator1/1, Relational Operator2/1, MinMax Running Resettable1/1
  Relational Operator2/1 -> MinMax Running Resettable1/2
  Constant/1 -> Relational Operator2/2
  If Action Subsystem/1(Out1) -> Sum/1  "picos6s"
  Sum/1 -> Product14/1
  Constant1/1 -> Sum/2

== system bluetooth/Subsystem/Electrocardiograma/FrecCardiaca/If Action Subsystem ==
  In1 : Inport
  Action Port : ActionPort  ActionPortLabel=if(u1 ==1)
  Out1 : Outport
  wires:
  In1/1 -> Out1/1

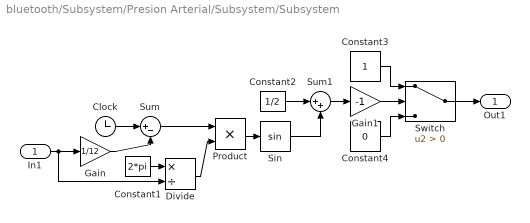
== system bluetooth/Subsystem/Presion Arterial/Subsystem/Subsystem ==
  In1 : Inport
  Clock : Clock
  Constant1 : Constant  Value=2*pi
  Constant2 : Constant  Value=1/2
  Constant3 : Constant
  Constant4 : Constant  Value=0
  Divide : Product  Inputs=*/
  Gain : Gain  Gain=1/12
  Gain1 : Gain  Gain=-1
  Product : Product
  Sin : Trigonometry
  Sum : Sum  Inputs=|+-
  Sum1 : Sum  Inputs=|++
  Switch : Switch  Criteria=u2 > Threshold
  Out1 : Outport
  wires:
  Constant1/1 -> Divide/1
  Divide/1 -> Product/2
  Constant2/1 -> Sum1/1
  Sum/1 -> Product/1
  Gain/1 -> Sum/2
  Constant3/1 -> Switch/1
  Sum1/1 -> Gain1/1
  Sin/1 -> Sum1/2
  Constant4/1 -> Switch/3
  Gain1/1 -> Switch/2
  Product/1 -> Sin/1
  In1/1 -> Divide/2, Gain/1
  Clock/1 -> Sum/1
  Switch/1 -> Out1/1

== system bluetooth/Subsystem/Respiracion/Subsystem/If Action Subsystem ==
  In1 : Inport
  Action Port : ActionPort  ActionPortLabel=if(u1 ==1)
  Out1 : Outport
  wires:
  In1/1 -> Out1/1

== matlab function bluetooth/caso de estudio ==
  data: u input; inTemp output; ECG output; presion output; CO2 output; ventilacion output
function [inTemp, ECG, presion, CO2, ventilacion] = fcn(u)
if u==0 %% normal
    %TEMP
    inTemp=1;
    %ECG
    alphaP= 0.6; %Valor de magnitud pico onda P
    alphaQ=-5;  %Valor de magnitud pico onda Q
    picoR=18;  %Valor de magnitud pico onda R
    alphaS=-7.5; %Valor de magnitud pico onda S
    alphaT=0.75*0.5; %Valor de magnitud pico onda T
    thetaP=pi/2;
    thetaQ=pi/12;
    thetaR=0;
    thetaS=pi/12;
    thetaT = 4*pi/6; % Angulo donde se ubica la onda T
    omegaECG=14; %Frecuencia angular ECG
    gananciaOut= 1.3;  %Valor para escalar salida del modelo    
    %%Presion
    Re0=0.0055222;Ra=0.025; Rlv=0.41279; Rv=0.02;
    Ce=1.69;Ca=2;Cv=15; c1=0.01; c2=4.0153; c3=0.000498;
    Ed=0.0655; Es0=0.57; epsilon=0.00001; A1=0.40341; 
    omega0=omegaECG;%8.37;
    %% CO2 85-92
    phi=92; %valor max de saturacion
    %tau1=0.2; %tiempo subida inspiracion
    %tau2=0.1; %tiempo subida espiracion
    d=1.5;  %Periodo /2
    
    %% Ventilación
    Ci=0.1;
    tf = d*2; %duración total del ciclo
    Vt=1.03;
    
elseif u==1  %%%%FIEBRE
    %Temp
    inTemp=1.05;
    %ECG
    alphaP= 0.6; %Valor de magnitud pico onda P
    alphaQ=-5;  %Valor de magnitud pico onda Q
    picoR=18;  %Valor de magnitud pico onda R
    alphaS=-7.5; %Valor de magnitud pico onda S
    alphaT=0.75*0.5; %Valor de magnitud pico onda T
    thetaP=pi/2;
    thetaQ=pi/12;
    thetaR=0;
    thetaS=pi/12;
    thetaT = 4*pi/6; % Angulo donde se ubica la onda T
    omegaECG=17; %Frecuencia angular ECG mayor a 180!!
    gananciaOut= 1.4; 
    %%Presion 85-42 aumenta para perder calor el cuero . No hipertension:
    %%esto depende de edad de peso
    Re0=0.0055222*1.3;Ra=0.025*1.3; Rlv=0.41279*1.3; Rv=0.02*1.3;
    Ce=1.69;Ca=2;Cv=15; c1=0.01; c2=4.0153; c3=0.000498;
    Ed=0.0655; Es0=0.57; epsilon=0.00001; A1=0.40341; 
    omega0=omegaECG;%8.37;
    %% CO2 (baja saturacion)
    phi=91; %valor max de saturacion
    %tau1=0.2; %tiempo subida inspiracion
    %tau2=0.1; %tiempo subida espiracion
    d=1.6;  %Periodo/2
    
    %% Ventilacion (mayor frec)
    Ci=0.1;
    tf = d*2;%0.8; %duración total del ciclo    Tiempo inspiratorio al aumnetar frec disminuye y por eso disminuye muy poco Co2
    Vt=1.03;
    
else %%%FRIO bradicardia! entre 60 y 100. Menor de 100 
    %Temp
    inTemp=0.95;
    %% ECG   
    alphaP= 0.6; %Valor de magnitud pico onda P
    alphaQ=-5;  %Valor de magnitud pico onda Q
    picoR=18;  %Valor de magnitud pico onda R
    alphaS=-7.5; %Valor de magnitud pico onda S
    alphaT=0.75*0.5; %Valor de magnitud pico onda T
    thetaP=pi/2;
    thetaQ=pi/12;
    thetaR=0;
    thetaS=pi/12;
    thetaT = 4*pi/6; % Angulo donde se ubica la onda T
    omegaECG=8; %Frecuencia angular ECG
    gananciaOut= 0.9;  %Valor para escalar salida del modelo 
    %%Presion disminuyen
    Re0=0.0055222;Ra=0.025; Rlv=0.41279; Rv=0.02;
    Ce=1.69;Ca=2;Cv=15; c1=0.01; c2=4.0153; c3=0.000498;
    Ed=0.0655; Es0=0.57; epsilon=0.00001; A1=0.40341; 
    omega0=omegaECG;%8.37;
    %% CO2 
    phi=80; %valor max de saturacion
    %tau1=0.2; %tiempo subida inspiracion
    %tau2=0.1; %tiempo subida espiracion
    d=2;  %Periodo
    %% Ventilacion
    Ci=0.1;
    tf = d*2; %duración total del ciclo
    Vt=1.03;
    
end
Tsys= 0.3333*2*pi/omega0;
Tdia= (1-0.3333)*2*pi/omega0;
Tpresion =Tsys+Tdia;

Ri=16.41;
ti=2;  %tiempo de inspiración
A = exp(ti/(Ri*Ci));
B= exp(tf/(Ri*Ci));
Pex= -(Vt*A)/(Ci*(A-B));
D= exp(-ti/(Ri*Ci));
Pset= Pex+(Vt/(D*(A-1)*Ci));

ECG=[alphaP,alphaQ, picoR, alphaS, alphaT,thetaP, thetaQ, thetaR, thetaS, thetaT, omegaECG,gananciaOut ];
presion=[Re0, Ra, Rlv, Rv, c1, c2, c3, Ed, Ce, Ca, Cv, Es0, epsilon, A1, omega0, Tpresion];
CO2=[phi,d];
ventilacion =[Pset, Pex, tf, Ci, Vt]; %falta condicion inicial y tiempos ti tf

== matlab function bluetooth/Heart rate converter ==
  data: HeartRate input; heartRateCharacteristic output; EnergyExpended input; RRInterval input
function heartRateCharacteristic = ConvertToHeartRateFormat(HeartRate, EnergyExpended, RRInterval)
flag = uint8(25);
heartRateCharacteristic = zeros(7,1,'uint8');
heartRateCharacteristic(1)= flag;
[lower, upper] = getBytes(HeartRate);
heartRateCharacteristic(2) = lower;
heartRateCharacteristic(3) = upper;
[lower, upper] = getBytes(EnergyExpended);
heartRateCharacteristic(4) = lower;
heartRateCharacteristic(5) = upper;
[lower, upper] = getBytes(RRInterval);
heartRateCharacteristic(6) = lower;
heartRateCharacteristic(7) = upper;
end

function [lower,upper] = getBytes(parameter)
h = dec2bin(parameter,16);
lower = bin2dec(h(9:16));
upper= bin2dec(h(1:8));
end

== matlab function bluetooth/InterpretHeartRateData1 ==
  data: u input; heartrate output; energyexpended output; rrinterval output
function [heartrate, energyexpended, rrinterval ] = InterpretHeartRateData(u)
flag = uint8(u(1));
heartrate = uint16(0);
energyexpended=uint16(0);
rrinterval = uint16(0);
b = bitget(flag,8:-1:1);

 if b(8) == 0
     format = uint8(2);
     heartrate = uint16(u(2));
 else
     format = uint8(3);
     heartrate = typecast([u(2) u(3)], 'uint16');
 end
 
 if b(5) == 1
     energy = uint8(2);
     energyexpended = typecast([u(format +1) u(format + 2)], 'uint16');
 else
     energy = uint8(0);
     energyexpended = uint16(0);
 end
 
 if b(4) == 1
     rrinterval = typecast([u(format +energy + 1) u(format + energy + 2)],'uint16');
 else
     rrinterval = uint16(0);
 end
end
